simulink model "Simulation_Robotinos"  (R2017b)
settings: Solver=FixedStepAuto  StartTime=0.0  StopTime=100.0  FixedStep=0.005  RelTol=1e-3
InitFcn:
  | dt=0.005;
libraries: simulink x15
(part 1 of 4)
settings Model: Creator=Robin  LastModifiedBy=Robin

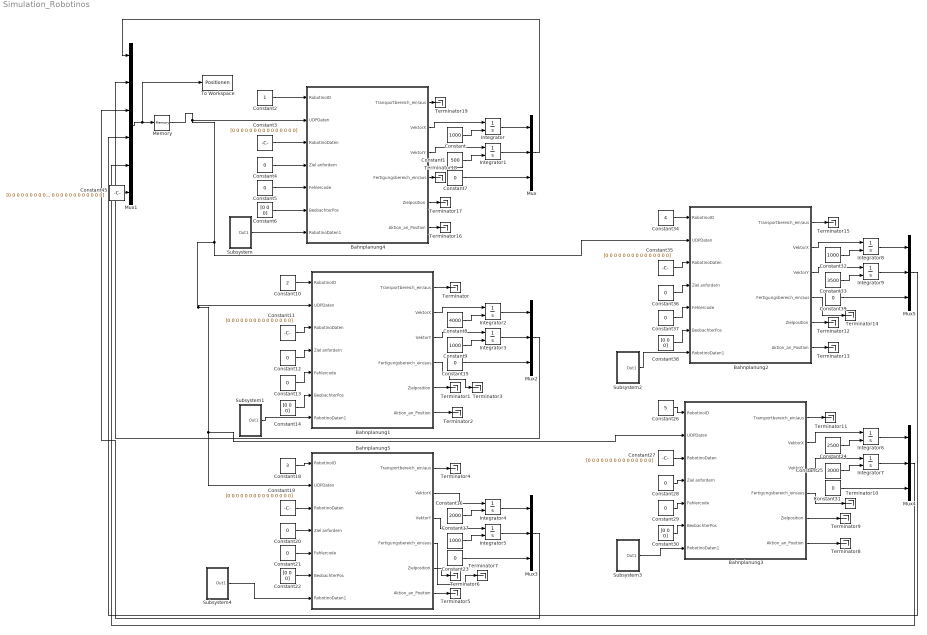
== system Simulation_Robotinos ==
  Bahnplanung1 : Subsystem
  Bahnplanung2 : Subsystem
  Bahnplanung3 : Subsystem
  Bahnplanung4 : Subsystem
  Bahnplanung5 : Subsystem
  Constant{,9,17,32} (4 alike) : Constant  Value=1000
  Constant1 : Constant  Value=500
  Constant10 : Constant  Value=2
  Constant{3,11,19,27,35} (5 alike) : Constant  Value=[0 0 0 0 0 0 0 0 0 0 0 0 0 0 0]
  Constant{4..5,7,12..13,15,20..21,23,28..29,31,36..37,39} (15 alike) : Constant  Value=0
  Constant{6,14,22,30,38} (5 alike) : Constant  Value=[0 0 0]
  Constant16 : Constant  Value=2000
  Constant18 : Constant  Value=3
  Constant2 : Constant
  Constant24 : Constant  Value=2500
  Constant25 : Constant  Value=3000
  Constant26 : Constant  Value=5
  Constant33 : Constant  Value=3500
  Constant34 : Constant  Value=4
  Constant45 : Constant  Value=[0 0 0 0 0 0 0 0 0 0 0 0 0 0 0 0 0 0 0 0 0 0 0 0 0 0 0 0 0 0 0 0 0 0 0 0 0 0 0 0 0]
  Constant8 : Constant  Value=4000
  Integrator{,1..9} (10 alike) : Integrator  InitialConditionSource=external
  Memory : Memory
  Mux{,2..5} (5 alike) : Mux  Inputs=3
  Mux1 : Mux  Inputs=6
  Subsystem : Subsystem
  Subsystem1 : Subsystem
  Subsystem2 : Subsystem
  Subsystem3 : Subsystem
  Subsystem4 : Subsystem
  Terminator{,1..19} (20 alike) : Terminator
  To Workspace : ToWorkspace  VariableName=Positionen  SaveFormat=Timeseries  SampleTime=-1
  wires:
  Bahnplanung4/3("VektorY ") -> Integrator1/1
  Bahnplanung4/2(VektorX) -> Integrator/1
  Constant/1 -> Integrator/2
  Constant1/1 -> Integrator1/2
  Integrator1/1 -> Mux/2
  Constant2/1 -> Bahnplanung4/1(RobotinoID)
  Constant3/1 -> Bahnplanung4/3(RobotinoDaten)
  Constant4/1 -> Bahnplanung4/4(Ziel anfordern)
  Constant5/1 -> Bahnplanung4/5(Fehlercode)
  Constant6/1 -> Bahnplanung4/6(BeobachterPos)
  Constant7/1 -> Mux/3
  Constant15/1 -> Mux2/3
  Constant13/1 -> Bahnplanung1/5(Fehlercode)
  Constant10/1 -> Bahnplanung1/1(RobotinoID)
  Constant8/1 -> Integrator2/2
  Bahnplanung1/3("VektorY ") -> Integrator3/1
  Constant12/1 -> Bahnplanung1/4(Ziel anfordern)
  Bahnplanung1/2(VektorX) -> Integrator2/1
  Constant9/1 -> Integrator3/2
  Integrator3/1 -> Mux2/2
  Integrator2/1 -> Mux2/1
  Constant11/1 -> Bahnplanung1/3(RobotinoDaten)
  Constant14/1 -> Bahnplanung1/6(BeobachterPos)
  Constant23/1 -> Mux3/3
  Constant21/1 -> Bahnplanung5/5(Fehlercode)
  Constant16/1 -> Integrator4/2
  Constant20/1 -> Bahnplanung5/4(Ziel anfordern)
  Constant17/1 -> Integrator5/2
  Integrator5/1 -> Mux3/2
  Integrator4/1 -> Mux3/1
  Constant19/1 -> Bahnplanung5/3(RobotinoDaten)
  Constant22/1 -> Bahnplanung5/6(BeobachterPos)
  Constant31/1 -> Mux4/3
  Constant29/1 -> Bahnplanung3/5(Fehlercode)
  Constant26/1 -> Bahnplanung3/1(RobotinoID)
  Constant24/1 -> Integrator6/2
  Constant28/1 -> Bahnplanung3/4(Ziel anfordern)
  Constant25/1 -> Integrator7/2
  Integrator7/1 -> Mux4/2
  Integrator6/1 -> Mux4/1
  Constant27/1 -> Bahnplanung3/3(RobotinoDaten)
  Constant30/1 -> Bahnplanung3/6(BeobachterPos)
  Constant39/1 -> Mux5/3
  Constant37/1 -> Bahnplanung2/5(Fehlercode)
  Constant34/1 -> Bahnplanung2/1(RobotinoID)
  Constant32/1 -> Integrator8/2
  Constant36/1 -> Bahnplanung2/4(Ziel anfordern)
  Memory/1 -> Bahnplanung2/2(UDPDaten), Bahnplanung1/2(UDPDaten), Bahnplanung5/2(UDPDaten), Bahnplanung3/2(UDPDaten), Bahnplanung4/2(UDPDaten)
  Constant33/1 -> Integrator9/2
  Integrator9/1 -> Mux5/2
  Integrator8/1 -> Mux5/1
  Constant35/1 -> Bahnplanung2/3(RobotinoDaten)
  Constant38/1 -> Bahnplanung2/6(BeobachterPos)
  Mux/1 -> Mux1/1
  Mux2/1 -> Mux1/2
  Mux3/1 -> Mux1/3
  Mux5/1 -> Mux1/4
  Mux4/1 -> Mux1/5
  Constant18/1 -> Bahnplanung5/1(RobotinoID)
  Subsystem4/1(Out1) -> Bahnplanung5/7(RobotinoDaten1)
  Subsystem1/1(Out1) -> Bahnplanung1/7(RobotinoDaten1)
  Subsystem3/1(Out1) -> Bahnplanung3/7(RobotinoDaten1)
  Subsystem2/1(Out1) -> Bahnplanung2/7(RobotinoDaten1)
  Mux1/1 -> To Workspace/1, Memory/1
  Constant45/1 -> Mux1/6
  Bahnplanung1/1(Transportbereich_ein/aus) -> Terminator/1
  Bahnplanung1/5(Zielposition) -> Terminator1/1
  Bahnplanung1/6(Aktion_an_Position) -> Terminator2/1
  Bahnplanung1/4(Fertigungsbereich_ein/aus) -> Terminator3/1
  Bahnplanung5/1(Transportbereich_ein/aus) -> Terminator4/1
  Bahnplanung5/6(Aktion_an_Position) -> Terminator5/1
  Bahnplanung5/5(Zielposition) -> Terminator6/1
  Bahnplanung5/4(Fertigungsbereich_ein/aus) -> Terminator7/1
  Bahnplanung3/5(Zielposition) -> Terminator9/1
  Bahnplanung3/6(Aktion_an_Position) -> Terminator8/1
  Bahnplanung3/4(Fertigungsbereich_ein/aus) -> Terminator10/1
  Bahnplanung3/1(Transportbereich_ein/aus) -> Terminator11/1
  Bahnplanung2/5(Zielposition) -> Terminator12/1
  Bahnplanung2/6(Aktion_an_Position) -> Terminator13/1
  Bahnplanung2/4(Fertigungsbereich_ein/aus) -> Terminator14/1
  Bahnplanung2/1(Transportbereich_ein/aus) -> Terminator15/1
  Bahnplanung4/6(Aktion_an_Position) -> Terminator16/1
  Bahnplanung4/5(Zielposition) -> Terminator17/1
  Bahnplanung4/4(Fertigungsbereich_ein/aus) -> Terminator18/1
  Bahnplanung4/1(Transportbereich_ein/aus) -> Terminator19/1
  Subsystem/1(Out1) -> Bahnplanung4/7(RobotinoDaten1)
  Integrator/1 -> Mux/1
  Bahnplanung5/2(VektorX) -> Integrator4/1
  Bahnplanung5/3("VektorY ") -> Integrator5/1
  Bahnplanung2/2(VektorX) -> Integrator8/1
  Bahnplanung2/3("VektorY ") -> Integrator9/1
  Bahnplanung3/2(VektorX) -> Integrator6/1
  Bahnplanung3/3("VektorY ") -> Integrator7/1

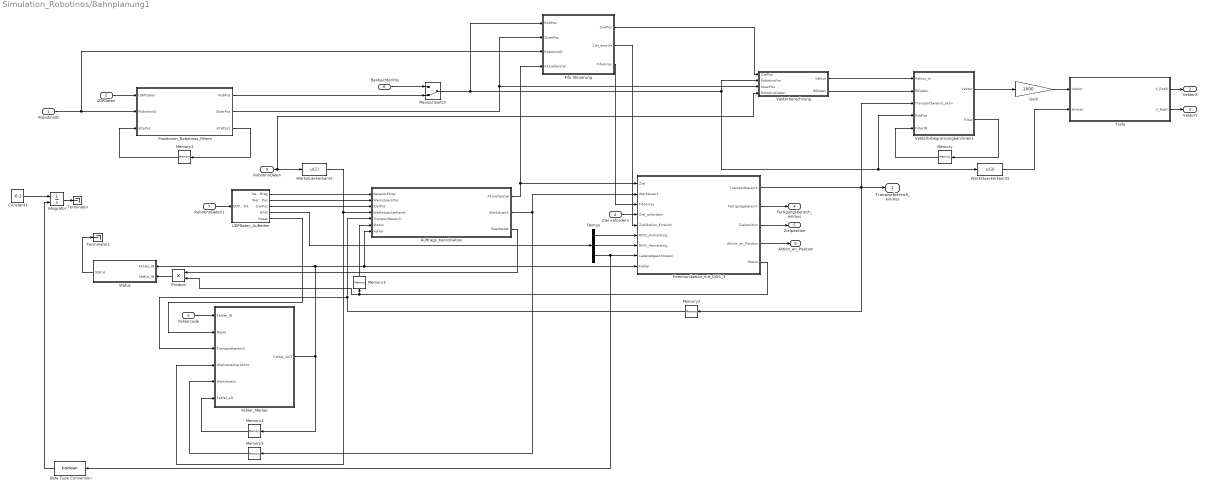
== system Simulation_Robotinos/Bahnplanung1 ==
  RobotinoID : Inport
  UDPDaten : Inport  Port=2  PortDimensions=56
  RobotinoDaten : Inport  Port=3
  Ziel anfordern : Inport  Port=4
  Fehlercode : Inport  Port=5
  BeobachterPos : Inport  Port=6
  RobotinoDaten1 : Inport  Port=7
  Auftrags_Koordination : Stateflow chart  TreatAsAtomicUnit=on
  Constant1 : Constant  Value=-0.2
  Data Type Conversion : DataTypeConversion  OutDataTypeStr=boolean
  Demux : Demux  Outputs=3
  Fehler_Merker : MATLAB Function  TreatAsAtomicUnit=on
  Fifo Steuerung : Subsystem
  Gain : Gain  Gain=-1000
  Integrator : Integrator  ExternalReset=rising  InitialCondition=100  LimitOutput=on  UpperSaturationLimit=100  LowerSaturationLimit=0
  Kommunikation_mit_GW1_3 : Stateflow chart  TreatAsAtomicUnit=on
  Manual Switch : ManualSwitch  CurrentSetting=0
  Memory{,1..5} (6 alike) : Memory
  Positionen_Robotinos_Filtern : MATLAB Function  TreatAsAtomicUnit=on
  Product : Product
  Status : MATLAB Function  TreatAsAtomicUnit=on
  Terminator : Terminator
  Terminator1 : Terminator
  Trafo : MATLAB Function  Tag=Transformation_Global_auf_lokal  TreatAsAtomicUnit=on
  UDPDaten_Aufteilen : Subsystem
  Vektorberechnung : Subsystem
  Vektorbrbegrenzungberchnen1 : MATLAB Function  TreatAsAtomicUnit=on
  Werkstueckerkannt : Fcn  Expr=u(1)
  Werkstueckerkannt1 : Fcn  Expr=u(3)
  Transportbereich_ein/aus : Outport
  VektorX : Outport  Port=2  OutDataTypeStr=double  PortDimensions=1
  "VektorY " : Outport  Port=3  OutDataTypeStr=double  PortDimensions=1
  Fertigungsbereich_ein/aus : Outport  Port=4
  Zielposition : Outport  Port=5
  Aktion_an_Position : Outport  Port=6
  wires:
  Vektorberechnung/2(IRDaten) -> Vektorbrbegrenzungberchnen1/2(IRDaten)
  Auftrags_Koordination/2(Werkstueck) -> Memory5/1, Kommunikation_mit_GW1_3/2(Werkstueck)
  Memory3/1 -> Auftrags_Koordination/6(Status)
  Kommunikation_mit_GW1_3/5(Status) -> Product/2, Memory3/1
  RobotinoID/1 -> Positionen_Robotinos_Filtern/2(RobotinoID), Fifo Steuerung/3(RobotinoID)
  UDPDaten/1 -> Positionen_Robotinos_Filtern/1(UDPDaten)
  Positionen_Robotinos_Filtern/2(StoerPos) -> Vektorberechnung/3(StoerPos), Fifo Steuerung/2(StoerPos)
  RobotinoDaten/1 -> Werkstueckerkannt/1, Vektorberechnung/4(RobotinoDaten)
  Kommunikation_mit_GW1_3/3(Zielposition) -> Zielposition/1
  Kommunikation_mit_GW1_3/4(Aktion_an_Position) -> Aktion_an_Position/1
  Kommunikation_mit_GW1_3/2(Fertigungsbereich) -> Fertigungsbereich_ein/aus/1
  Kommunikation_mit_GW1_3/1(Transportbereich) -> Transportbereich_ein/aus/1, Vektorbrbegrenzungberchnen1/3(Transportbereich_aktiv), Memory2/1
  RobotinoDaten1/1 -> UDPDaten_Aufteilen/1(UDP_GW1)
  UDPDaten_Aufteilen/2(WerkstueckPos) -> Auftrags_Koordination/2(WerkstueckPos)
  UDPDaten_Aufteilen/3(ZielPos) -> Auftrags_Koordination/3(ZielPos)
  Auftrags_Koordination/1(AktuellesZiel) -> Fifo Steuerung/4(AktuellesZiel), Kommunikation_mit_GW1_3/1(Ziel)
  UDPDaten_Aufteilen/1(NeuerAuftrag) -> Auftrags_Koordination/1(NeuerAuftrag)
  Werkstueckerkannt/1 -> Auftrags_Koordination/4(Werkstueckerkannt), Fehler_Merker/4(Werkstueckerkannt)
  Vektorbrbegrenzungberchnen1/1(Vektor) -> Gain/1
  Gain/1 -> Trafo/1(Vektor)
  Manual Switch/1 -> Vektorberechnung/2(RobotinoPos), Vektorbrbegrenzungberchnen1/4(RobPos), Werkstueckerkannt1/1, Fifo Steuerung/1(RobPos)
  Vektorberechnung/1(Vektor) -> Vektorbrbegrenzungberchnen1/1(Vektor_In)
  Fifo Steuerung/1(ZielPos) -> Vektorberechnung/1(ZielPos)
  Memory2/1 -> Auftrags_Koordination/5(Transportbereich), Fehler_Merker/3(Transportbereich)
  Positionen_Robotinos_Filtern/1(RobPos) -> Manual Switch/2
  Trafo/1(V_RobX) -> VektorX/1
  Trafo/2(V_RobY) -> "VektorY "/1
  BeobachterPos/1 -> Manual Switch/1
  Werkstueckerkannt1/1 -> Trafo/2(Winkel)
  Auftrags_Koordination/3(Bearbeitet) -> Product/1
  UDPDaten_Aufteilen/4(RFID) -> Demux/1
  Fifo Steuerung/3("FifoArray ") -> Kommunikation_mit_GW1_3/3(FifoArray)
  Ziel anfordern/1 -> Kommunikation_mit_GW1_3/4(Ziel_anfordern)
  Fifo Steuerung/2(Ziel_ereciht) -> Kommunikation_mit_GW1_3/5(ZielStation_Erreicht)
  Demux/1 -> Kommunikation_mit_GW1_3/6(RFID_Anmeldung)
  Demux/2 -> Kommunikation_mit_GW1_3/7(RFID_Abmeldung)
  Vektorbrbegrenzungberchnen1/2(Filter) -> Memory/1
  Memory/1 -> Vektorbrbegrenzungberchnen1/5(FilterIN)
  Positionen_Robotinos_Filtern/3(altePos1) -> Memory1/1
  Memory1/1 -> Positionen_Robotinos_Filtern/3(altePos)
  Demux/3 -> Kommunikation_mit_GW1_3/8(Ladenabgeschlossen), Data Type Conversion/1
  Fehlercode/1 -> Fehler_Merker/1(Fehler_IN)
  Constant1/1 -> Integrator/1
  Data Type Conversion/1 -> Integrator/2
  Product/1 -> Status/2(Status_IN)
  UDPDaten_Aufteilen/5(Reset) -> Fehler_Merker/2(Reset)
  Memory4/1 -> Fehler_Merker/6(Fehler_alt)
  Fehler_Merker/1(Fehler_OUT) -> Status/1(Fehler_IN), Kommunikation_mit_GW1_3/9(Fehler), Auftrags_Koordination/7(Fehler), Memory4/1
  Memory5/1 -> Fehler_Merker/5(Werkstueck)
  Integrator/1 -> Terminator/1
  Status/1(Status) -> Terminator1/1

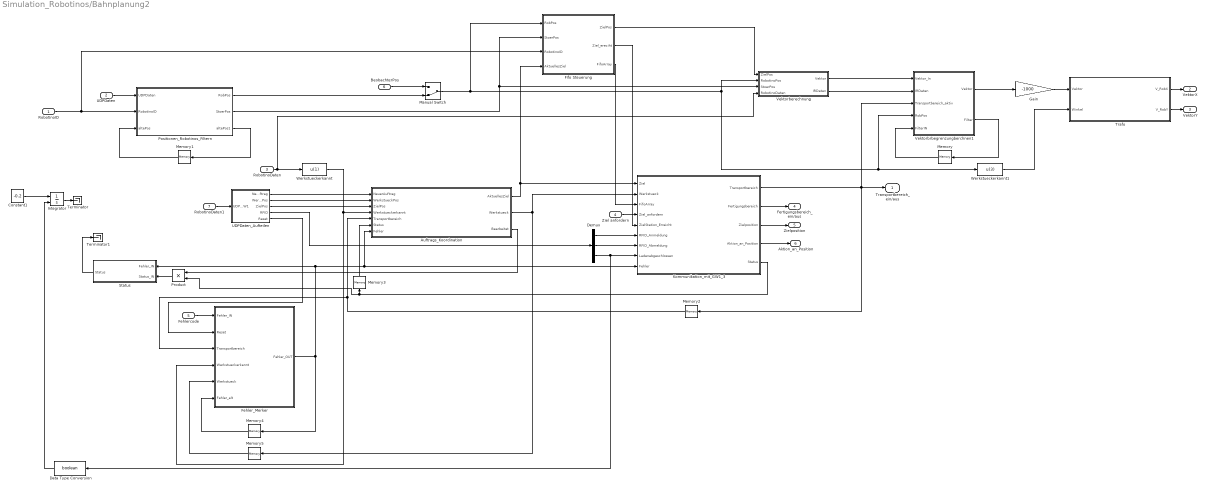
== system Simulation_Robotinos/Bahnplanung2 ==
  RobotinoID : Inport
  UDPDaten : Inport  Port=2  PortDimensions=56
  RobotinoDaten : Inport  Port=3
  Ziel anfordern : Inport  Port=4
  Fehlercode : Inport  Port=5
  BeobachterPos : Inport  Port=6
  RobotinoDaten1 : Inport  Port=7
  Auftrags_Koordination : Stateflow chart  TreatAsAtomicUnit=on
  Constant1 : Constant  Value=-0.2
  Data Type Conversion : DataTypeConversion  OutDataTypeStr=boolean
  Demux : Demux  Outputs=3
  Fehler_Merker : MATLAB Function  TreatAsAtomicUnit=on
  Fifo Steuerung : Subsystem
  Gain : Gain  Gain=-1000
  Integrator : Integrator  ExternalReset=rising  InitialCondition=100  LimitOutput=on  UpperSaturationLimit=100  LowerSaturationLimit=0
  Kommunikation_mit_GW1_3 : Stateflow chart  TreatAsAtomicUnit=on
  Manual Switch : ManualSwitch  CurrentSetting=0
  Memory{,1..5} (6 alike) : Memory
  Positionen_Robotinos_Filtern : MATLAB Function  TreatAsAtomicUnit=on
  Product : Product
  Status : MATLAB Function  TreatAsAtomicUnit=on
  Terminator : Terminator
  Terminator1 : Terminator
  Trafo : MATLAB Function  Tag=Transformation_Global_auf_lokal  TreatAsAtomicUnit=on
  UDPDaten_Aufteilen : Subsystem
  Vektorberechnung : Subsystem
  Vektorbrbegrenzungberchnen1 : MATLAB Function  TreatAsAtomicUnit=on
  Werkstueckerkannt : Fcn  Expr=u(1)
  Werkstueckerkannt1 : Fcn  Expr=u(3)
  Transportbereich_ein/aus : Outport
  VektorX : Outport  Port=2  OutDataTypeStr=double  PortDimensions=1
  "VektorY " : Outport  Port=3  OutDataTypeStr=double  PortDimensions=1
  Fertigungsbereich_ein/aus : Outport  Port=4
  Zielposition : Outport  Port=5
  Aktion_an_Position : Outport  Port=6
  wires:
  Status/1(Status) -> Terminator1/1
  Integrator/1 -> Terminator/1
  Memory5/1 -> Fehler_Merker/5(Werkstueck)
  Fehler_Merker/1(Fehler_OUT) -> Memory4/1, Auftrags_Koordination/7(Fehler), Kommunikation_mit_GW1_3/9(Fehler), Status/1(Fehler_IN)
  Memory4/1 -> Fehler_Merker/6(Fehler_alt)
  UDPDaten_Aufteilen/5(Reset) -> Fehler_Merker/2(Reset)
  Product/1 -> Status/2(Status_IN)
  Data Type Conversion/1 -> Integrator/2
  Constant1/1 -> Integrator/1
  Fehlercode/1 -> Fehler_Merker/1(Fehler_IN)
  Demux/3 -> Data Type Conversion/1, Kommunikation_mit_GW1_3/8(Ladenabgeschlossen)
  Memory1/1 -> Positionen_Robotinos_Filtern/3(altePos)
  Positionen_Robotinos_Filtern/3(altePos1) -> Memory1/1
  Memory/1 -> Vektorbrbegrenzungberchnen1/5(FilterIN)
  Vektorbrbegrenzungberchnen1/2(Filter) -> Memory/1
  Demux/2 -> Kommunikation_mit_GW1_3/7(RFID_Abmeldung)
  Demux/1 -> Kommunikation_mit_GW1_3/6(RFID_Anmeldung)
  Fifo Steuerung/2(Ziel_ereciht) -> Kommunikation_mit_GW1_3/5(ZielStation_Erreicht)
  Ziel anfordern/1 -> Kommunikation_mit_GW1_3/4(Ziel_anfordern)
  Fifo Steuerung/3("FifoArray ") -> Kommunikation_mit_GW1_3/3(FifoArray)
  UDPDaten_Aufteilen/4(RFID) -> Demux/1
  Auftrags_Koordination/3(Bearbeitet) -> Product/1
  Werkstueckerkannt1/1 -> Trafo/2(Winkel)
  BeobachterPos/1 -> Manual Switch/1
  Trafo/2(V_RobY) -> "VektorY "/1
  Trafo/1(V_RobX) -> VektorX/1
  Positionen_Robotinos_Filtern/1(RobPos) -> Manual Switch/2
  Memory2/1 -> Fehler_Merker/3(Transportbereich), Auftrags_Koordination/5(Transportbereich)
  Fifo Steuerung/1(ZielPos) -> Vektorberechnung/1(ZielPos)
  Vektorberechnung/1(Vektor) -> Vektorbrbegrenzungberchnen1/1(Vektor_In)
  Manual Switch/1 -> Fifo Steuerung/1(RobPos), Werkstueckerkannt1/1, Vektorbrbegrenzungberchnen1/4(RobPos), Vektorberechnung/2(RobotinoPos)
  Gain/1 -> Trafo/1(Vektor)
  Vektorbrbegrenzungberchnen1/1(Vektor) -> Gain/1
  Werkstueckerkannt/1 -> Fehler_Merker/4(Werkstueckerkannt), Auftrags_Koordination/4(Werkstueckerkannt)
  UDPDaten_Aufteilen/1(NeuerAuftrag) -> Auftrags_Koordination/1(NeuerAuftrag)
  Auftrags_Koordination/1(AktuellesZiel) -> Kommunikation_mit_GW1_3/1(Ziel), Fifo Steuerung/4(AktuellesZiel)
  UDPDaten_Aufteilen/3(ZielPos) -> Auftrags_Koordination/3(ZielPos)
  UDPDaten_Aufteilen/2(WerkstueckPos) -> Auftrags_Koordination/2(WerkstueckPos)
  RobotinoDaten1/1 -> UDPDaten_Aufteilen/1(UDP_GW1)
  Kommunikation_mit_GW1_3/1(Transportbereich) -> Memory2/1, Vektorbrbegrenzungberchnen1/3(Transportbereich_aktiv), Transportbereich_ein/aus/1
  Kommunikation_mit_GW1_3/2(Fertigungsbereich) -> Fertigungsbereich_ein/aus/1
  Kommunikation_mit_GW1_3/4(Aktion_an_Position) -> Aktion_an_Position/1
  Kommunikation_mit_GW1_3/3(Zielposition) -> Zielposition/1
  RobotinoDaten/1 -> Vektorberechnung/4(RobotinoDaten), Werkstueckerkannt/1
  Positionen_Robotinos_Filtern/2(StoerPos) -> Fifo Steuerung/2(StoerPos), Vektorberechnung/3(StoerPos)
  UDPDaten/1 -> Positionen_Robotinos_Filtern/1(UDPDaten)
  RobotinoID/1 -> Fifo Steuerung/3(RobotinoID), Positionen_Robotinos_Filtern/2(RobotinoID)
  Kommunikation_mit_GW1_3/5(Status) -> Memory3/1, Product/2
  Memory3/1 -> Auftrags_Koordination/6(Status)
  Auftrags_Koordination/2(Werkstueck) -> Kommunikation_mit_GW1_3/2(Werkstueck), Memory5/1
  Vektorberechnung/2(IRDaten) -> Vektorbrbegrenzungberchnen1/2(IRDaten)

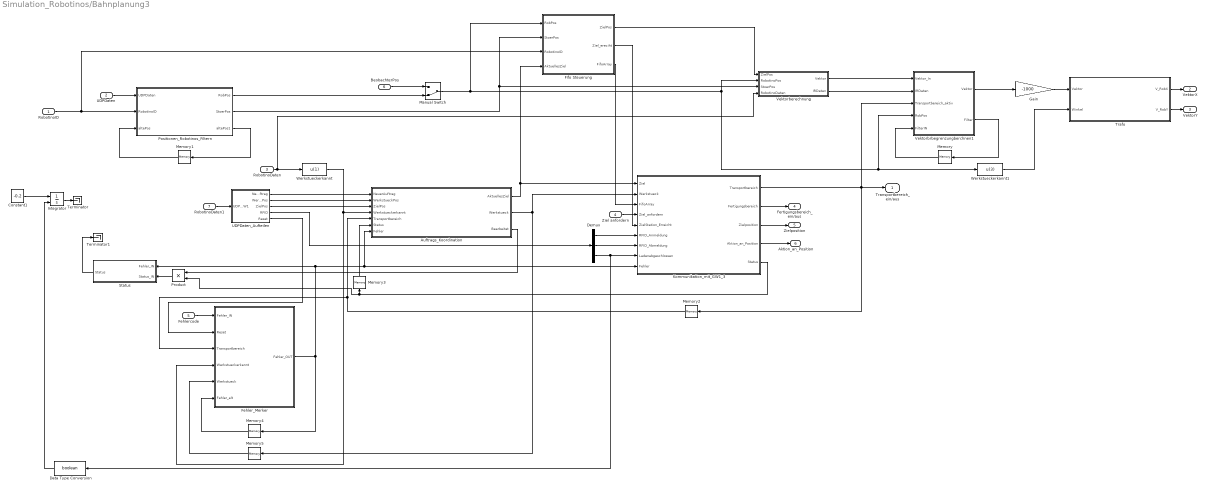
== system Simulation_Robotinos/Bahnplanung3 ==
  RobotinoID : Inport
  UDPDaten : Inport  Port=2  PortDimensions=56
  RobotinoDaten : Inport  Port=3
  Ziel anfordern : Inport  Port=4
  Fehlercode : Inport  Port=5
  BeobachterPos : Inport  Port=6
  RobotinoDaten1 : Inport  Port=7
  Auftrags_Koordination : Stateflow chart  TreatAsAtomicUnit=on
  Constant1 : Constant  Value=-0.2
  Data Type Conversion : DataTypeConversion  OutDataTypeStr=boolean
  Demux : Demux  Outputs=3
  Fehler_Merker : MATLAB Function  TreatAsAtomicUnit=on
  Fifo Steuerung : Subsystem
  Gain : Gain  Gain=-1000
  Integrator : Integrator  ExternalReset=rising  InitialCondition=100  LimitOutput=on  UpperSaturationLimit=100  LowerSaturationLimit=0
  Kommunikation_mit_GW1_3 : Stateflow chart  TreatAsAtomicUnit=on
  Manual Switch : ManualSwitch  CurrentSetting=0
  Memory{,1..5} (6 alike) : Memory
  Positionen_Robotinos_Filtern : MATLAB Function  TreatAsAtomicUnit=on
  Product : Product
  Status : MATLAB Function  TreatAsAtomicUnit=on
  Terminator : Terminator
  Terminator1 : Terminator
  Trafo : MATLAB Function  Tag=Transformation_Global_auf_lokal  TreatAsAtomicUnit=on
  UDPDaten_Aufteilen : Subsystem
  Vektorberechnung : Subsystem
  Vektorbrbegrenzungberchnen1 : MATLAB Function  TreatAsAtomicUnit=on
  Werkstueckerkannt : Fcn  Expr=u(1)
  Werkstueckerkannt1 : Fcn  Expr=u(3)
  Transportbereich_ein/aus : Outport
  VektorX : Outport  Port=2  OutDataTypeStr=double  PortDimensions=1
  "VektorY " : Outport  Port=3  OutDataTypeStr=double  PortDimensions=1
  Fertigungsbereich_ein/aus : Outport  Port=4
  Zielposition : Outport  Port=5
  Aktion_an_Position : Outport  Port=6
  wires:
  Vektorberechnung/2(IRDaten) -> Vektorbrbegrenzungberchnen1/2(IRDaten)
  Auftrags_Koordination/2(Werkstueck) -> Memory5/1, Kommunikation_mit_GW1_3/2(Werkstueck)
  Memory3/1 -> Auftrags_Koordination/6(Status)
  Kommunikation_mit_GW1_3/5(Status) -> Product/2, Memory3/1
  RobotinoID/1 -> Positionen_Robotinos_Filtern/2(RobotinoID), Fifo Steuerung/3(RobotinoID)
  UDPDaten/1 -> Positionen_Robotinos_Filtern/1(UDPDaten)
  Positionen_Robotinos_Filtern/2(StoerPos) -> Vektorberechnung/3(StoerPos), Fifo Steuerung/2(StoerPos)
  RobotinoDaten/1 -> Werkstueckerkannt/1, Vektorberechnung/4(RobotinoDaten)
  Kommunikation_mit_GW1_3/3(Zielposition) -> Zielposition/1
  Kommunikation_mit_GW1_3/4(Aktion_an_Position) -> Aktion_an_Position/1
  Kommunikation_mit_GW1_3/2(Fertigungsbereich) -> Fertigungsbereich_ein/aus/1
  Kommunikation_mit_GW1_3/1(Transportbereich) -> Transportbereich_ein/aus/1, Vektorbrbegrenzungberchnen1/3(Transportbereich_aktiv), Memory2/1
  RobotinoDaten1/1 -> UDPDaten_Aufteilen/1(UDP_GW1)
  UDPDaten_Aufteilen/2(WerkstueckPos) -> Auftrags_Koordination/2(WerkstueckPos)
  UDPDaten_Aufteilen/3(ZielPos) -> Auftrags_Koordination/3(ZielPos)
  Auftrags_Koordination/1(AktuellesZiel) -> Fifo Steuerung/4(AktuellesZiel), Kommunikation_mit_GW1_3/1(Ziel)
  UDPDaten_Aufteilen/1(NeuerAuftrag) -> Auftrags_Koordination/1(NeuerAuftrag)
  Werkstueckerkannt/1 -> Auftrags_Koordination/4(Werkstueckerkannt), Fehler_Merker/4(Werkstueckerkannt)
  Vektorbrbegrenzungberchnen1/1(Vektor) -> Gain/1
  Gain/1 -> Trafo/1(Vektor)
  Manual Switch/1 -> Vektorberechnung/2(RobotinoPos), Vektorbrbegrenzungberchnen1/4(RobPos), Werkstueckerkannt1/1, Fifo Steuerung/1(RobPos)
  Vektorberechnung/1(Vektor) -> Vektorbrbegrenzungberchnen1/1(Vektor_In)
  Fifo Steuerung/1(ZielPos) -> Vektorberechnung/1(ZielPos)
  Memory2/1 -> Auftrags_Koordination/5(Transportbereich), Fehler_Merker/3(Transportbereich)
  Positionen_Robotinos_Filtern/1(RobPos) -> Manual Switch/2
  Trafo/1(V_RobX) -> VektorX/1
  Trafo/2(V_RobY) -> "VektorY "/1
  BeobachterPos/1 -> Manual Switch/1
  Werkstueckerkannt1/1 -> Trafo/2(Winkel)
  Auftrags_Koordination/3(Bearbeitet) -> Product/1
  UDPDaten_Aufteilen/4(RFID) -> Demux/1
  Fifo Steuerung/3("FifoArray ") -> Kommunikation_mit_GW1_3/3(FifoArray)
  Ziel anfordern/1 -> Kommunikation_mit_GW1_3/4(Ziel_anfordern)
  Fifo Steuerung/2(Ziel_ereciht) -> Kommunikation_mit_GW1_3/5(ZielStation_Erreicht)
  Demux/1 -> Kommunikation_mit_GW1_3/6(RFID_Anmeldung)
  Demux/2 -> Kommunikation_mit_GW1_3/7(RFID_Abmeldung)
  Vektorbrbegrenzungberchnen1/2(Filter) -> Memory/1
  Memory/1 -> Vektorbrbegrenzungberchnen1/5(FilterIN)
  Positionen_Robotinos_Filtern/3(altePos1) -> Memory1/1
  Memory1/1 -> Positionen_Robotinos_Filtern/3(altePos)
  Demux/3 -> Kommunikation_mit_GW1_3/8(Ladenabgeschlossen), Data Type Conversion/1
  Fehlercode/1 -> Fehler_Merker/1(Fehler_IN)
  Constant1/1 -> Integrator/1
  Data Type Conversion/1 -> Integrator/2
  Product/1 -> Status/2(Status_IN)
  UDPDaten_Aufteilen/5(Reset) -> Fehler_Merker/2(Reset)
  Memory4/1 -> Fehler_Merker/6(Fehler_alt)
  Fehler_Merker/1(Fehler_OUT) -> Status/1(Fehler_IN), Kommunikation_mit_GW1_3/9(Fehler), Auftrags_Koordination/7(Fehler), Memory4/1
  Memory5/1 -> Fehler_Merker/5(Werkstueck)
  Integrator/1 -> Terminator/1
  Status/1(Status) -> Terminator1/1

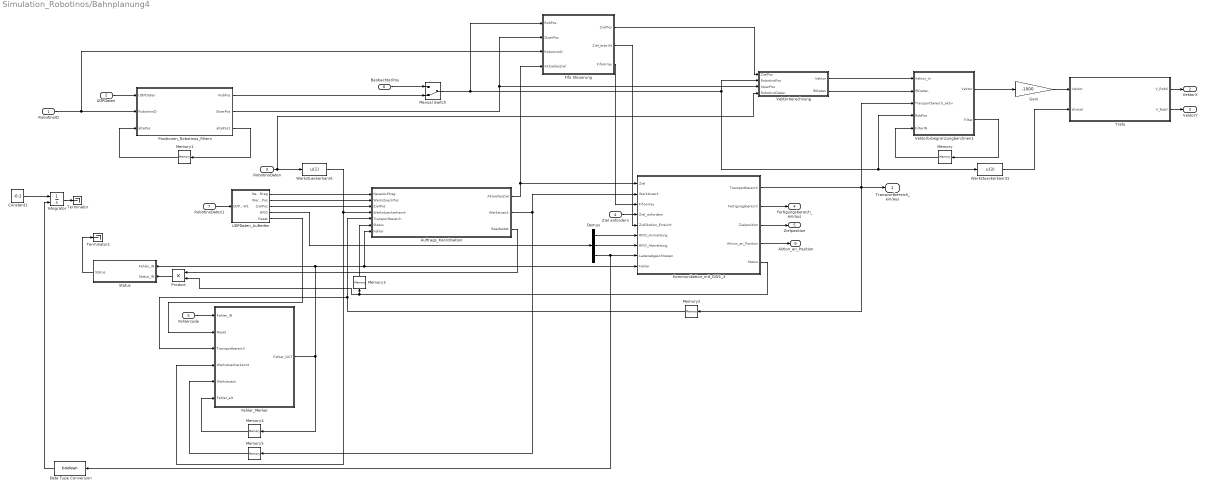
== system Simulation_Robotinos/Bahnplanung4 ==
  RobotinoID : Inport
  UDPDaten : Inport  Port=2  PortDimensions=56
  RobotinoDaten : Inport  Port=3
  Ziel anfordern : Inport  Port=4
  Fehlercode : Inport  Port=5
  BeobachterPos : Inport  Port=6
  RobotinoDaten1 : Inport  Port=7
  Auftrags_Koordination : Stateflow chart  TreatAsAtomicUnit=on
  Constant1 : Constant  Value=-0.2
  Data Type Conversion : DataTypeConversion  OutDataTypeStr=boolean
  Demux : Demux  Outputs=3
  Fehler_Merker : MATLAB Function  TreatAsAtomicUnit=on
  Fifo Steuerung : Subsystem
  Gain : Gain  Gain=-1000
  Integrator : Integrator  ExternalReset=rising  InitialCondition=100  LimitOutput=on  UpperSaturationLimit=100  LowerSaturationLimit=0
  Kommunikation_mit_GW1_3 : Stateflow chart  TreatAsAtomicUnit=on
  Manual Switch : ManualSwitch  CurrentSetting=0
  Memory{,1..5} (6 alike) : Memory
  Positionen_Robotinos_Filtern : MATLAB Function  TreatAsAtomicUnit=on
  Product : Product
  Status : MATLAB Function  TreatAsAtomicUnit=on
  Terminator : Terminator
  Terminator1 : Terminator
  Trafo : MATLAB Function  Tag=Transformation_Global_auf_lokal  TreatAsAtomicUnit=on
  UDPDaten_Aufteilen : Subsystem
  Vektorberechnung : Subsystem
  Vektorbrbegrenzungberchnen1 : MATLAB Function  TreatAsAtomicUnit=on
  Werkstueckerkannt : Fcn  Expr=u(1)
  Werkstueckerkannt1 : Fcn  Expr=u(3)
  Transportbereich_ein/aus : Outport
  VektorX : Outport  Port=2  OutDataTypeStr=double  PortDimensions=1
  "VektorY " : Outport  Port=3  OutDataTypeStr=double  PortDimensions=1
  Fertigungsbereich_ein/aus : Outport  Port=4
  Zielposition : Outport  Port=5
  Aktion_an_Position : Outport  Port=6
  wires:
  Status/1(Status) -> Terminator1/1
  Integrator/1 -> Terminator/1
  Memory5/1 -> Fehler_Merker/5(Werkstueck)
  Fehler_Merker/1(Fehler_OUT) -> Memory4/1, Auftrags_Koordination/7(Fehler), Kommunikation_mit_GW1_3/9(Fehler), Status/1(Fehler_IN)
  Memory4/1 -> Fehler_Merker/6(Fehler_alt)
  UDPDaten_Aufteilen/5(Reset) -> Fehler_Merker/2(Reset)
  Product/1 -> Status/2(Status_IN)
  Data Type Conversion/1 -> Integrator/2
  Constant1/1 -> Integrator/1
  Fehlercode/1 -> Fehler_Merker/1(Fehler_IN)
  Demux/3 -> Data Type Conversion/1, Kommunikation_mit_GW1_3/8(Ladenabgeschlossen)
  Memory1/1 -> Positionen_Robotinos_Filtern/3(altePos)
  Positionen_Robotinos_Filtern/3(altePos1) -> Memory1/1
  Memory/1 -> Vektorbrbegrenzungberchnen1/5(FilterIN)
  Vektorbrbegrenzungberchnen1/2(Filter) -> Memory/1
  Demux/2 -> Kommunikation_mit_GW1_3/7(RFID_Abmeldung)
  Demux/1 -> Kommunikation_mit_GW1_3/6(RFID_Anmeldung)
  Fifo Steuerung/2(Ziel_ereciht) -> Kommunikation_mit_GW1_3/5(ZielStation_Erreicht)
  Ziel anfordern/1 -> Kommunikation_mit_GW1_3/4(Ziel_anfordern)
  Fifo Steuerung/3("FifoArray ") -> Kommunikation_mit_GW1_3/3(FifoArray)
  UDPDaten_Aufteilen/4(RFID) -> Demux/1
  Auftrags_Koordination/3(Bearbeitet) -> Product/1
  Werkstueckerkannt1/1 -> Trafo/2(Winkel)
  BeobachterPos/1 -> Manual Switch/1
  Trafo/2(V_RobY) -> "VektorY "/1
  Trafo/1(V_RobX) -> VektorX/1
  Positionen_Robotinos_Filtern/1(RobPos) -> Manual Switch/2
  Memory2/1 -> Fehler_Merker/3(Transportbereich), Auftrags_Koordination/5(Transportbereich)
  Fifo Steuerung/1(ZielPos) -> Vektorberechnung/1(ZielPos)
  Vektorberechnung/1(Vektor) -> Vektorbrbegrenzungberchnen1/1(Vektor_In)
  Manual Switch/1 -> Fifo Steuerung/1(RobPos), Werkstueckerkannt1/1, Vektorbrbegrenzungberchnen1/4(RobPos), Vektorberechnung/2(RobotinoPos)
  Gain/1 -> Trafo/1(Vektor)
  Vektorbrbegrenzungberchnen1/1(Vektor) -> Gain/1
  Werkstueckerkannt/1 -> Fehler_Merker/4(Werkstueckerkannt), Auftrags_Koordination/4(Werkstueckerkannt)
  UDPDaten_Aufteilen/1(NeuerAuftrag) -> Auftrags_Koordination/1(NeuerAuftrag)
  Auftrags_Koordination/1(AktuellesZiel) -> Kommunikation_mit_GW1_3/1(Ziel), Fifo Steuerung/4(AktuellesZiel)
  UDPDaten_Aufteilen/3(ZielPos) -> Auftrags_Koordination/3(ZielPos)
  UDPDaten_Aufteilen/2(WerkstueckPos) -> Auftrags_Koordination/2(WerkstueckPos)
  RobotinoDaten1/1 -> UDPDaten_Aufteilen/1(UDP_GW1)
  Kommunikation_mit_GW1_3/1(Transportbereich) -> Memory2/1, Vektorbrbegrenzungberchnen1/3(Transportbereich_aktiv), Transportbereich_ein/aus/1
  Kommunikation_mit_GW1_3/2(Fertigungsbereich) -> Fertigungsbereich_ein/aus/1
  Kommunikation_mit_GW1_3/4(Aktion_an_Position) -> Aktion_an_Position/1
  Kommunikation_mit_GW1_3/3(Zielposition) -> Zielposition/1
  RobotinoDaten/1 -> Vektorberechnung/4(RobotinoDaten), Werkstueckerkannt/1
  Positionen_Robotinos_Filtern/2(StoerPos) -> Fifo Steuerung/2(StoerPos), Vektorberechnung/3(StoerPos)
  UDPDaten/1 -> Positionen_Robotinos_Filtern/1(UDPDaten)
  RobotinoID/1 -> Fifo Steuerung/3(RobotinoID), Positionen_Robotinos_Filtern/2(RobotinoID)
  Kommunikation_mit_GW1_3/5(Status) -> Memory3/1, Product/2
  Memory3/1 -> Auftrags_Koordination/6(Status)
  Auftrags_Koordination/2(Werkstueck) -> Kommunikation_mit_GW1_3/2(Werkstueck), Memory5/1
  Vektorberechnung/2(IRDaten) -> Vektorbrbegrenzungberchnen1/2(IRDaten)

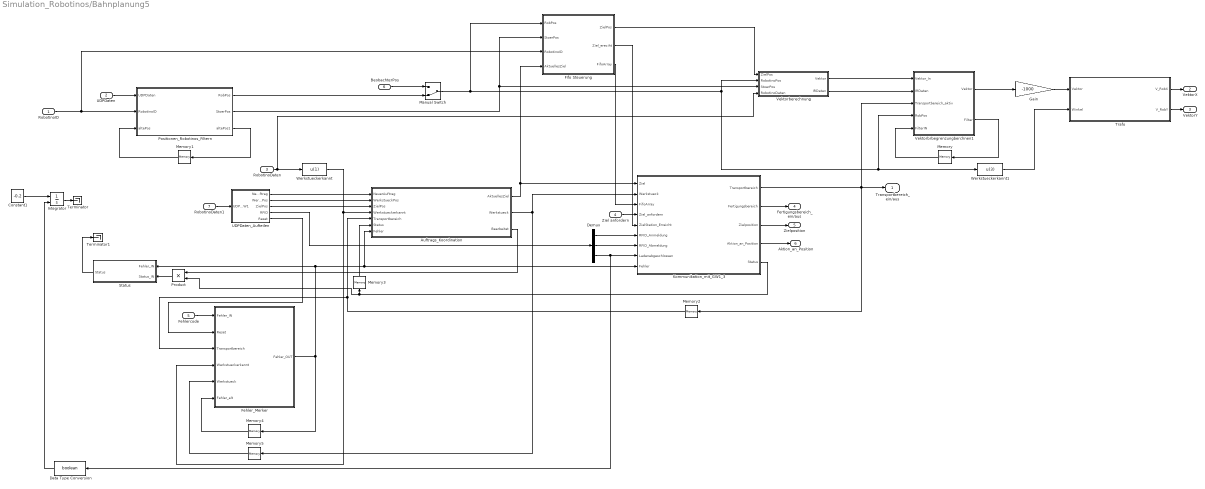
== system Simulation_Robotinos/Bahnplanung5 ==
  RobotinoID : Inport
  UDPDaten : Inport  Port=2  PortDimensions=56
  RobotinoDaten : Inport  Port=3
  Ziel anfordern : Inport  Port=4
  Fehlercode : Inport  Port=5
  BeobachterPos : Inport  Port=6
  RobotinoDaten1 : Inport  Port=7
  Auftrags_Koordination : Stateflow chart  TreatAsAtomicUnit=on
  Constant1 : Constant  Value=-0.2
  Data Type Conversion : DataTypeConversion  OutDataTypeStr=boolean
  Demux : Demux  Outputs=3
  Fehler_Merker : MATLAB Function  TreatAsAtomicUnit=on
  Fifo Steuerung : Subsystem
  Gain : Gain  Gain=-1000
  Integrator : Integrator  ExternalReset=rising  InitialCondition=100  LimitOutput=on  UpperSaturationLimit=100  LowerSaturationLimit=0
  Kommunikation_mit_GW1_3 : Stateflow chart  TreatAsAtomicUnit=on
  Manual Switch : ManualSwitch  CurrentSetting=0
  Memory{,1..5} (6 alike) : Memory
  Positionen_Robotinos_Filtern : MATLAB Function  TreatAsAtomicUnit=on
  Product : Product
  Status : MATLAB Function  TreatAsAtomicUnit=on
  Terminator : Terminator
  Terminator1 : Terminator
  Trafo : MATLAB Function  Tag=Transformation_Global_auf_lokal  TreatAsAtomicUnit=on
  UDPDaten_Aufteilen : Subsystem
  Vektorberechnung : Subsystem
  Vektorbrbegrenzungberchnen1 : MATLAB Function  TreatAsAtomicUnit=on
  Werkstueckerkannt : Fcn  Expr=u(1)
  Werkstueckerkannt1 : Fcn  Expr=u(3)
  Transportbereich_ein/aus : Outport
  VektorX : Outport  Port=2  OutDataTypeStr=double  PortDimensions=1
  "VektorY " : Outport  Port=3  OutDataTypeStr=double  PortDimensions=1
  Fertigungsbereich_ein/aus : Outport  Port=4
  Zielposition : Outport  Port=5
  Aktion_an_Position : Outport  Port=6
  wires:
  Status/1(Status) -> Terminator1/1
  Integrator/1 -> Terminator/1
  Memory5/1 -> Fehler_Merker/5(Werkstueck)
  Fehler_Merker/1(Fehler_OUT) -> Memory4/1, Auftrags_Koordination/7(Fehler), Kommunikation_mit_GW1_3/9(Fehler), Status/1(Fehler_IN)
  Memory4/1 -> Fehler_Merker/6(Fehler_alt)
  UDPDaten_Aufteilen/5(Reset) -> Fehler_Merker/2(Reset)
  Product/1 -> Status/2(Status_IN)
  Data Type Conversion/1 -> Integrator/2
  Constant1/1 -> Integrator/1
  Fehlercode/1 -> Fehler_Merker/1(Fehler_IN)
  Demux/3 -> Data Type Conversion/1, Kommunikation_mit_GW1_3/8(Ladenabgeschlossen)
  Memory1/1 -> Positionen_Robotinos_Filtern/3(altePos)
  Positionen_Robotinos_Filtern/3(altePos1) -> Memory1/1
  Memory/1 -> Vektorbrbegrenzungberchnen1/5(FilterIN)
  Vektorbrbegrenzungberchnen1/2(Filter) -> Memory/1
  Demux/2 -> Kommunikation_mit_GW1_3/7(RFID_Abmeldung)
  Demux/1 -> Kommunikation_mit_GW1_3/6(RFID_Anmeldung)
  Fifo Steuerung/2(Ziel_ereciht) -> Kommunikation_mit_GW1_3/5(ZielStation_Erreicht)
  Ziel anfordern/1 -> Kommunikation_mit_GW1_3/4(Ziel_anfordern)
  Fifo Steuerung/3("FifoArray ") -> Kommunikation_mit_GW1_3/3(FifoArray)
  UDPDaten_Aufteilen/4(RFID) -> Demux/1
  Auftrags_Koordination/3(Bearbeitet) -> Product/1
  Werkstueckerkannt1/1 -> Trafo/2(Winkel)
  BeobachterPos/1 -> Manual Switch/1
  Trafo/2(V_RobY) -> "VektorY "/1
  Trafo/1(V_RobX) -> VektorX/1
  Positionen_Robotinos_Filtern/1(RobPos) -> Manual Switch/2
  Memory2/1 -> Fehler_Merker/3(Transportbereich), Auftrags_Koordination/5(Transportbereich)
  Fifo Steuerung/1(ZielPos) -> Vektorberechnung/1(ZielPos)
  Vektorberechnung/1(Vektor) -> Vektorbrbegrenzungberchnen1/1(Vektor_In)
  Manual Switch/1 -> Fifo Steuerung/1(RobPos), Werkstueckerkannt1/1, Vektorbrbegrenzungberchnen1/4(RobPos), Vektorberechnung/2(RobotinoPos)
  Gain/1 -> Trafo/1(Vektor)
  Vektorbrbegrenzungberchnen1/1(Vektor) -> Gain/1
  Werkstueckerkannt/1 -> Fehler_Merker/4(Werkstueckerkannt), Auftrags_Koordination/4(Werkstueckerkannt)
  UDPDaten_Aufteilen/1(NeuerAuftrag) -> Auftrags_Koordination/1(NeuerAuftrag)
  Auftrags_Koordination/1(AktuellesZiel) -> Kommunikation_mit_GW1_3/1(Ziel), Fifo Steuerung/4(AktuellesZiel)
  UDPDaten_Aufteilen/3(ZielPos) -> Auftrags_Koordination/3(ZielPos)
  UDPDaten_Aufteilen/2(WerkstueckPos) -> Auftrags_Koordination/2(WerkstueckPos)
  RobotinoDaten1/1 -> UDPDaten_Aufteilen/1(UDP_GW1)
  Kommunikation_mit_GW1_3/1(Transportbereich) -> Memory2/1, Vektorbrbegrenzungberchnen1/3(Transportbereich_aktiv), Transportbereich_ein/aus/1
  Kommunikation_mit_GW1_3/2(Fertigungsbereich) -> Fertigungsbereich_ein/aus/1
  Kommunikation_mit_GW1_3/4(Aktion_an_Position) -> Aktion_an_Position/1
  Kommunikation_mit_GW1_3/3(Zielposition) -> Zielposition/1
  RobotinoDaten/1 -> Vektorberechnung/4(RobotinoDaten), Werkstueckerkannt/1
  Positionen_Robotinos_Filtern/2(StoerPos) -> Fifo Steuerung/2(StoerPos), Vektorberechnung/3(StoerPos)
  UDPDaten/1 -> Positionen_Robotinos_Filtern/1(UDPDaten)
  RobotinoID/1 -> Fifo Steuerung/3(RobotinoID), Positionen_Robotinos_Filtern/2(RobotinoID)
  Kommunikation_mit_GW1_3/5(Status) -> Memory3/1, Product/2
  Memory3/1 -> Auftrags_Koordination/6(Status)
  Auftrags_Koordination/2(Werkstueck) -> Kommunikation_mit_GW1_3/2(Werkstueck), Memory5/1
  Vektorberechnung/2(IRDaten) -> Vektorbrbegrenzungberchnen1/2(IRDaten)

== system Simulation_Robotinos/Subsystem ==
  Constant44 : Constant  Value=[0 0 ]
  Constant46 : Constant  Value=[2 1 1 1 7 1]
  Mux6 : Mux  Inputs=3
  Step : Step  Time=0.01  SampleTime=0
  Out1 : Outport
  wires:
  Constant46/1 -> Mux6/3
  Constant44/1 -> Mux6/1
  Mux6/1 -> Out1/1
  Step/1 -> Mux6/2

== system Simulation_Robotinos/Subsystem1 ==
  Constant44 : Constant  Value=[0 0 ]
  Constant46 : Constant  Value=[2 1 1 1 7 1]
  Mux6 : Mux  Inputs=3
  Step : Step  Time=0.01  SampleTime=0
  Out1 : Outport
  wires:
  Step/1 -> Mux6/2
  Mux6/1 -> Out1/1
  Constant44/1 -> Mux6/1
  Constant46/1 -> Mux6/3

== system Simulation_Robotinos/Subsystem2 ==
  Constant44 : Constant  Value=[0 0 ]
  Constant46 : Constant  Value=[2 1 1 1 7 1]
  Mux6 : Mux  Inputs=3
  Step : Step  Time=0.01  SampleTime=0
  Out1 : Outport
  wires:
  Constant46/1 -> Mux6/3
  Constant44/1 -> Mux6/1
  Mux6/1 -> Out1/1
  Step/1 -> Mux6/2

== system Simulation_Robotinos/Subsystem3 ==
  Constant44 : Constant  Value=[0 0 ]
  Constant46 : Constant  Value=[2 1 1 1 7 1]
  Mux6 : Mux  Inputs=3
  Step : Step  Time=0.01  SampleTime=0
  Out1 : Outport
  wires:
  Step/1 -> Mux6/2
  Mux6/1 -> Out1/1
  Constant44/1 -> Mux6/1
  Constant46/1 -> Mux6/3

== system Simulation_Robotinos/Subsystem4 ==
  Constant44 : Constant  Value=[0 0 ]
  Constant46 : Constant  Value=[2 1 1 1 7 1]
  Mux6 : Mux  Inputs=3
  Step : Step  Time=0.01  SampleTime=0
  Out1 : Outport
  wires:
  Constant46/1 -> Mux6/3
  Constant44/1 -> Mux6/1
  Mux6/1 -> Out1/1
  Step/1 -> Mux6/2

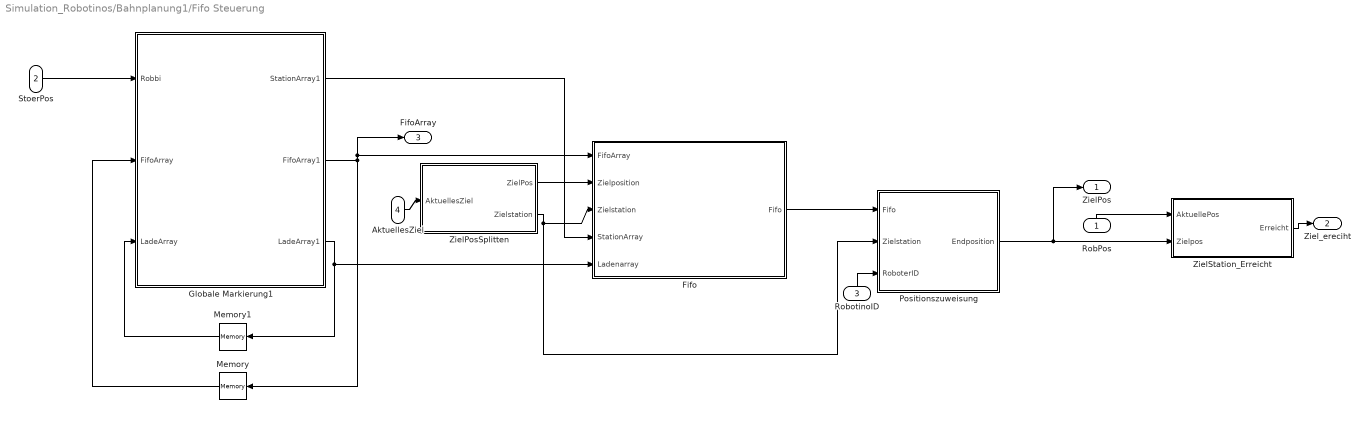
== system Simulation_Robotinos/Bahnplanung1/Fifo Steuerung ==
  RobPos : Inport  PortDimensions=3
  StoerPos : Inport  Port=2  PortDimensions=15
  RobotinoID : Inport  Port=3
  AktuellesZiel : Inport  Port=4
  Fifo : Stateflow chart  TreatAsAtomicUnit=on
  Globale Markierung1 : MATLAB Function  TreatAsAtomicUnit=on
  Memory : Memory
  Memory1 : Memory
  Positionszuweisung : MATLAB Function  TreatAsAtomicUnit=on
  ZielPosSplitten : MATLAB Function  TreatAsAtomicUnit=on
  ZielStation_Erreicht : MATLAB Function  TreatAsAtomicUnit=on
  ZielPos : Outport  PortDimensions=[1 2]
  Ziel_ereciht : Outport  Port=2
  "FifoArray " : Outport  Port=3
  wires:
  RobotinoID/1 -> Positionszuweisung/3(RoboterID)
  RobPos/1 -> ZielStation_Erreicht/1(AktuellePos)
  StoerPos/1 -> Globale Markierung1/1(Robbi)
  AktuellesZiel/1 -> ZielPosSplitten/1(AktuellesZiel)
  Positionszuweisung/1(Endposition) -> ZielStation_Erreicht/2(Zielpos), ZielPos/1
  Globale Markierung1/1(StationArray1) -> Fifo/4(StationArray)
  ZielPosSplitten/1(ZielPos) -> Fifo/2(Zielposition)
  ZielPosSplitten/2(Zielstation) -> Positionszuweisung/2(Zielstation), Fifo/3(Zielstation)
  Memory/1 -> Globale Markierung1/2(FifoArray)
  Globale Markierung1/3(LadeArray1) -> Fifo/5(Ladenarray), Memory1/1
  Memory1/1 -> Globale Markierung1/3(LadeArray)
  ZielStation_Erreicht/1(Erreicht) -> Ziel_ereciht/1
  Fifo/1(Fifo) -> Positionszuweisung/1(Fifo)
  Globale Markierung1/2(FifoArray1) -> "FifoArray "/1, Fifo/1(FifoArray), Memory/1

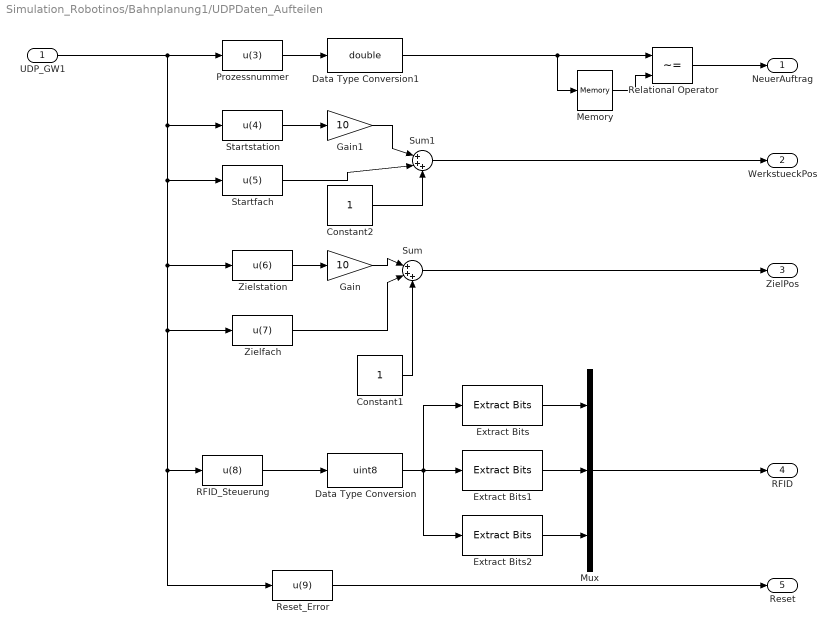
== system Simulation_Robotinos/Bahnplanung1/UDPDaten_Aufteilen ==
  UDP_GW1 : Inport
  Constant1 : Constant
  Constant2 : Constant
  Data Type Conversion : DataTypeConversion  OutDataTypeStr=uint8
  Data Type Conversion1 : DataTypeConversion  OutDataTypeStr=double
  Extract Bits : simulink/Logic and Bit Operations/Extract Bits  bitsToExtract=Range of bits  numBits=8  bitIdxRange=[0]  outScalingMode=Treat bit field as an integer
      settings: SourceProductName=Simulink
  Extract Bits1 : simulink/Logic and Bit Operations/Extract Bits  bitsToExtract=Range of bits  numBits=8  bitIdxRange=[1]  outScalingMode=Treat bit field as an integer
      settings: SourceProductName=Simulink
  Extract Bits2 : simulink/Logic and Bit Operations/Extract Bits  bitsToExtract=Range of bits  numBits=8  bitIdxRange=[2]  outScalingMode=Treat bit field as an integer
      settings: SourceProductName=Simulink
  Gain : Gain  Gain=10
  Gain1 : Gain  Gain=10
  Memory : Memory
  Mux : Mux  Inputs=3
  Prozessnummer : Fcn  Expr=u(3)
  RFID_Steuerung : Fcn  Expr=u(8)
  Relational Operator : RelationalOperator  Operator=~=  OutDataTypeStr=boolean  RndMeth=Nearest
  Reset_Error : Fcn  Expr=u(9)
  Startfach : Fcn  Expr=u(5)
  Startstation : Fcn  Expr=u(4)
  Sum : Sum  Inputs=|+++
  Sum1 : Sum  Inputs=|+++
  Zielfach : Fcn  Expr=u(7)
  Zielstation : Fcn  Expr=u(6)
  NeuerAuftrag : Outport
  WerkstueckPos : Outport  Port=2
  ZielPos : Outport  Port=3
  RFID : Outport  Port=4
  Reset : Outport  Port=5
  wires:
  Zielfach/1 -> Sum/2
  Gain/1 -> Sum/1
  Zielstation/1 -> Gain/1
  UDP_GW1/1 -> Prozessnummer/1, Startstation/1, Startfach/1, Zielstation/1, RFID_Steuerung/1, Reset_Error/1, Zielfach/1
  Sum1/1 -> WerkstueckPos/1
  Startfach/1 -> Sum1/2
  Gain1/1 -> Sum1/1
  Constant2/1 -> Sum1/3
  Startstation/1 -> Gain1/1
  Constant1/1 -> Sum/3
  Sum/1 -> ZielPos/1
  Relational Operator/1 -> NeuerAuftrag/1
  RFID_Steuerung/1 -> Data Type Conversion/1
  Data Type Conversion/1 -> Extract Bits2/1, Extract Bits1/1, Extract Bits/1
  Data Type Conversion1/1 -> Relational Operator/1, Memory/1
  Memory/1 -> Relational Operator/2
  Extract Bits1/1 -> Mux/2
  Mux/1 -> RFID/1
  Prozessnummer/1 -> Data Type Conversion1/1
  Extract Bits/1 -> Mux/1
  Extract Bits2/1 -> Mux/3
  Reset_Error/1 -> Reset/1

== system Simulation_Robotinos/Bahnplanung1/Vektorberechnung ==
  ZielPos : Inport
  RobotinoPos : Inport  Port=2
  StoerPos : Inport  Port=3
  RobotinoDaten : Inport  Port=4  PortDimensions=15
  AusweichVektorBerechnung : MATLAB Function  TreatAsAtomicUnit=on
  Ausweichmanoever : MATLAB Function  TreatAsAtomicUnit=on
  FahrendeRobotinosErkennen : MATLAB Function  TreatAsAtomicUnit=on
  Gain1 : Gain  Gain=-1
  IR_Daten_Erfassen : MATLAB Function  TreatAsAtomicUnit=on
  Memory : Memory
  Transport Delay : TransportDelay
  Vektorberechnung : MATLAB Function  TreatAsAtomicUnit=on
  Vektor : Outport
  IRDaten : Outport  Port=2
  wires:
  RobotinoPos/1 -> IR_Daten_Erfassen/2(RobPos), Vektorberechnung/3(RobotinoPos), AusweichVektorBerechnung/3(RobotinoPos), Ausweichmanoever/1(RobotinoPos)
  RobotinoDaten/1 -> IR_Daten_Erfassen/1(RobotinoDaten)
  StoerPos/1 -> Vektorberechnung/1(StoerPos), Ausweichmanoever/2(StoerPos), Transport Delay/1, FahrendeRobotinosErkennen/1(Stoerpos)
  ZielPos/1 -> Vektorberechnung/5(ZielPos), AusweichVektorBerechnung/2(ZielPos)
  Ausweichmanoever/1(Ausweich) -> AusweichVektorBerechnung/4(Ausweichwert)
  Vektorberechnung/1(Vektor) -> Gain1/1, AusweichVektorBerechnung/5(Vektor_In)
  Gain1/1 -> Ausweichmanoever/3(Vektor)
  IR_Daten_Erfassen/1(IRWerte) -> Vektorberechnung/2(IRWerte), IRDaten/1
  AusweichVektorBerechnung/1(Vektor) -> Vektor/1
  Vektorberechnung/2(Zone) -> Memory/1, AusweichVektorBerechnung/1(Zone)
  FahrendeRobotinosErkennen/1(Robotinofaehrt) -> Vektorberechnung/4(RobotinoFaehrt)
  Transport Delay/1 -> FahrendeRobotinosErkennen/2(Stoeralt)
  Memory/1 -> Vektorberechnung/6(AlteZone)

== system Simulation_Robotinos/Bahnplanung2/Fifo Steuerung ==
  RobPos : Inport  PortDimensions=3
  StoerPos : Inport  Port=2  PortDimensions=15
  RobotinoID : Inport  Port=3
  AktuellesZiel : Inport  Port=4
  Fifo : Stateflow chart  TreatAsAtomicUnit=on
  Globale Markierung1 : MATLAB Function  TreatAsAtomicUnit=on
  Memory : Memory
  Memory1 : Memory
  Positionszuweisung : MATLAB Function  TreatAsAtomicUnit=on
  ZielPosSplitten : MATLAB Function  TreatAsAtomicUnit=on
  ZielStation_Erreicht : MATLAB Function  TreatAsAtomicUnit=on
  ZielPos : Outport  PortDimensions=[1 2]
  Ziel_ereciht : Outport  Port=2
  "FifoArray " : Outport  Port=3
  wires:
  Globale Markierung1/2(FifoArray1) -> Memory/1, Fifo/1(FifoArray), "FifoArray "/1
  Fifo/1(Fifo) -> Positionszuweisung/1(Fifo)
  ZielStation_Erreicht/1(Erreicht) -> Ziel_ereciht/1
  Memory1/1 -> Globale Markierung1/3(LadeArray)
  Globale Markierung1/3(LadeArray1) -> Memory1/1, Fifo/5(Ladenarray)
  Memory/1 -> Globale Markierung1/2(FifoArray)
  ZielPosSplitten/2(Zielstation) -> Fifo/3(Zielstation), Positionszuweisung/2(Zielstation)
  ZielPosSplitten/1(ZielPos) -> Fifo/2(Zielposition)
  Globale Markierung1/1(StationArray1) -> Fifo/4(StationArray)
  Positionszuweisung/1(Endposition) -> ZielPos/1, ZielStation_Erreicht/2(Zielpos)
  AktuellesZiel/1 -> ZielPosSplitten/1(AktuellesZiel)
  StoerPos/1 -> Globale Markierung1/1(Robbi)
  RobPos/1 -> ZielStation_Erreicht/1(AktuellePos)
  RobotinoID/1 -> Positionszuweisung/3(RoboterID)

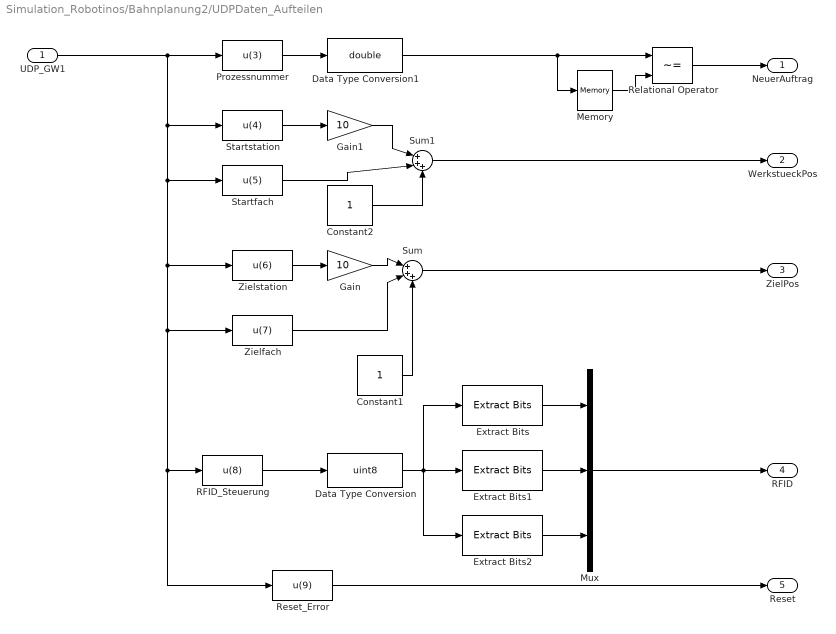
== system Simulation_Robotinos/Bahnplanung2/UDPDaten_Aufteilen ==
  UDP_GW1 : Inport
  Constant1 : Constant
  Constant2 : Constant
  Data Type Conversion : DataTypeConversion  OutDataTypeStr=uint8
  Data Type Conversion1 : DataTypeConversion  OutDataTypeStr=double
  Extract Bits : simulink/Logic and Bit Operations/Extract Bits  bitsToExtract=Range of bits  numBits=8  bitIdxRange=[0]  outScalingMode=Treat bit field as an integer
      settings: SourceProductName=Simulink
  Extract Bits1 : simulink/Logic and Bit Operations/Extract Bits  bitsToExtract=Range of bits  numBits=8  bitIdxRange=[1]  outScalingMode=Treat bit field as an integer
      settings: SourceProductName=Simulink
  Extract Bits2 : simulink/Logic and Bit Operations/Extract Bits  bitsToExtract=Range of bits  numBits=8  bitIdxRange=[2]  outScalingMode=Treat bit field as an integer
      settings: SourceProductName=Simulink
  Gain : Gain  Gain=10
  Gain1 : Gain  Gain=10
  Memory : Memory
  Mux : Mux  Inputs=3
  Prozessnummer : Fcn  Expr=u(3)
  RFID_Steuerung : Fcn  Expr=u(8)
  Relational Operator : RelationalOperator  Operator=~=  OutDataTypeStr=boolean  RndMeth=Nearest
  Reset_Error : Fcn  Expr=u(9)
  Startfach : Fcn  Expr=u(5)
  Startstation : Fcn  Expr=u(4)
  Sum : Sum  Inputs=|+++
  Sum1 : Sum  Inputs=|+++
  Zielfach : Fcn  Expr=u(7)
  Zielstation : Fcn  Expr=u(6)
  NeuerAuftrag : Outport
  WerkstueckPos : Outport  Port=2
  ZielPos : Outport  Port=3
  RFID : Outport  Port=4
  Reset : Outport  Port=5
  wires:
  Reset_Error/1 -> Reset/1
  Extract Bits2/1 -> Mux/3
  Extract Bits/1 -> Mux/1
  Prozessnummer/1 -> Data Type Conversion1/1
  Mux/1 -> RFID/1
  Extract Bits1/1 -> Mux/2
  Memory/1 -> Relational Operator/2
  Data Type Conversion1/1 -> Memory/1, Relational Operator/1
  Data Type Conversion/1 -> Extract Bits/1, Extract Bits1/1, Extract Bits2/1
  RFID_Steuerung/1 -> Data Type Conversion/1
  Relational Operator/1 -> NeuerAuftrag/1
  Sum/1 -> ZielPos/1
  Constant1/1 -> Sum/3
  Startstation/1 -> Gain1/1
  Constant2/1 -> Sum1/3
  Gain1/1 -> Sum1/1
  Startfach/1 -> Sum1/2
  Sum1/1 -> WerkstueckPos/1
  UDP_GW1/1 -> Zielfach/1, Reset_Error/1, RFID_Steuerung/1, Zielstation/1, Startfach/1, Startstation/1, Prozessnummer/1
  Zielstation/1 -> Gain/1
  Gain/1 -> Sum/1
  Zielfach/1 -> Sum/2

== system Simulation_Robotinos/Bahnplanung2/Vektorberechnung ==
  ZielPos : Inport
  RobotinoPos : Inport  Port=2
  StoerPos : Inport  Port=3
  RobotinoDaten : Inport  Port=4  PortDimensions=15
  AusweichVektorBerechnung : MATLAB Function  TreatAsAtomicUnit=on
  Ausweichmanoever : MATLAB Function  TreatAsAtomicUnit=on
  FahrendeRobotinosErkennen : MATLAB Function  TreatAsAtomicUnit=on
  Gain1 : Gain  Gain=-1
  IR_Daten_Erfassen : MATLAB Function  TreatAsAtomicUnit=on
  Memory : Memory
  Transport Delay : TransportDelay
  Vektorberechnung : MATLAB Function  TreatAsAtomicUnit=on
  Vektor : Outport
  IRDaten : Outport  Port=2
  wires:
  Memory/1 -> Vektorberechnung/6(AlteZone)
  Transport Delay/1 -> FahrendeRobotinosErkennen/2(Stoeralt)
  FahrendeRobotinosErkennen/1(Robotinofaehrt) -> Vektorberechnung/4(RobotinoFaehrt)
  Vektorberechnung/2(Zone) -> AusweichVektorBerechnung/1(Zone), Memory/1
  AusweichVektorBerechnung/1(Vektor) -> Vektor/1
  IR_Daten_Erfassen/1(IRWerte) -> IRDaten/1, Vektorberechnung/2(IRWerte)
  Gain1/1 -> Ausweichmanoever/3(Vektor)
  Vektorberechnung/1(Vektor) -> AusweichVektorBerechnung/5(Vektor_In), Gain1/1
  Ausweichmanoever/1(Ausweich) -> AusweichVektorBerechnung/4(Ausweichwert)
  ZielPos/1 -> AusweichVektorBerechnung/2(ZielPos), Vektorberechnung/5(ZielPos)
  StoerPos/1 -> FahrendeRobotinosErkennen/1(Stoerpos), Transport Delay/1, Ausweichmanoever/2(StoerPos), Vektorberechnung/1(StoerPos)
  RobotinoDaten/1 -> IR_Daten_Erfassen/1(RobotinoDaten)
  RobotinoPos/1 -> Ausweichmanoever/1(RobotinoPos), AusweichVektorBerechnung/3(RobotinoPos), Vektorberechnung/3(RobotinoPos), IR_Daten_Erfassen/2(RobPos)

== system Simulation_Robotinos/Bahnplanung3/Fifo Steuerung ==
  RobPos : Inport  PortDimensions=3
  StoerPos : Inport  Port=2  PortDimensions=15
  RobotinoID : Inport  Port=3
  AktuellesZiel : Inport  Port=4
  Fifo : Stateflow chart  TreatAsAtomicUnit=on
  Globale Markierung1 : MATLAB Function  TreatAsAtomicUnit=on
  Memory : Memory
  Memory1 : Memory
  Positionszuweisung : MATLAB Function  TreatAsAtomicUnit=on
  ZielPosSplitten : MATLAB Function  TreatAsAtomicUnit=on
  ZielStation_Erreicht : MATLAB Function  TreatAsAtomicUnit=on
  ZielPos : Outport  PortDimensions=[1 2]
  Ziel_ereciht : Outport  Port=2
  "FifoArray " : Outport  Port=3
  wires:
  RobotinoID/1 -> Positionszuweisung/3(RoboterID)
  RobPos/1 -> ZielStation_Erreicht/1(AktuellePos)
  StoerPos/1 -> Globale Markierung1/1(Robbi)
  AktuellesZiel/1 -> ZielPosSplitten/1(AktuellesZiel)
  Positionszuweisung/1(Endposition) -> ZielStation_Erreicht/2(Zielpos), ZielPos/1
  Globale Markierung1/1(StationArray1) -> Fifo/4(StationArray)
  ZielPosSplitten/1(ZielPos) -> Fifo/2(Zielposition)
  ZielPosSplitten/2(Zielstation) -> Positionszuweisung/2(Zielstation), Fifo/3(Zielstation)
  Memory/1 -> Globale Markierung1/2(FifoArray)
  Globale Markierung1/3(LadeArray1) -> Fifo/5(Ladenarray), Memory1/1
  Memory1/1 -> Globale Markierung1/3(LadeArray)
  ZielStation_Erreicht/1(Erreicht) -> Ziel_ereciht/1
  Fifo/1(Fifo) -> Positionszuweisung/1(Fifo)
  Globale Markierung1/2(FifoArray1) -> "FifoArray "/1, Fifo/1(FifoArray), Memory/1

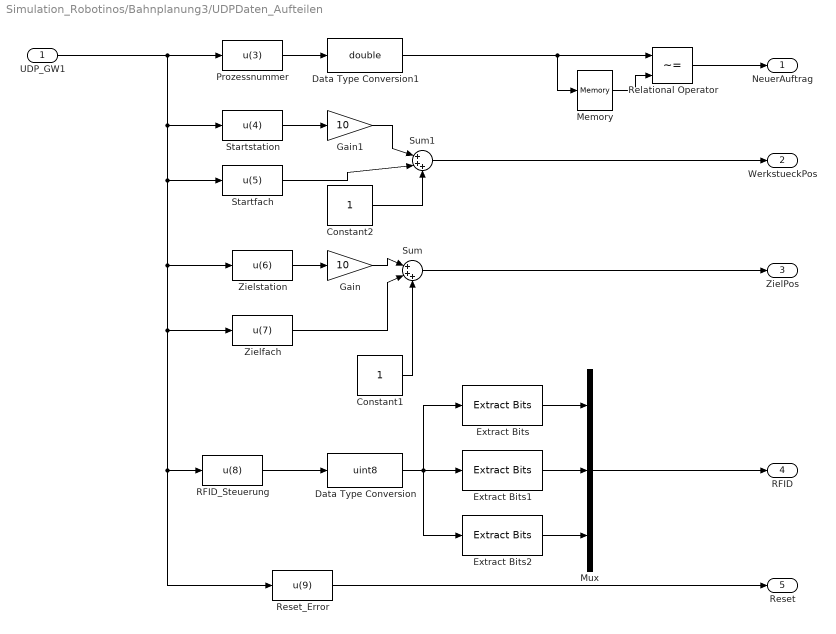
== system Simulation_Robotinos/Bahnplanung3/UDPDaten_Aufteilen ==
  UDP_GW1 : Inport
  Constant1 : Constant
  Constant2 : Constant
  Data Type Conversion : DataTypeConversion  OutDataTypeStr=uint8
  Data Type Conversion1 : DataTypeConversion  OutDataTypeStr=double
  Extract Bits : simulink/Logic and Bit Operations/Extract Bits  bitsToExtract=Range of bits  numBits=8  bitIdxRange=[0]  outScalingMode=Treat bit field as an integer
      settings: SourceProductName=Simulink
  Extract Bits1 : simulink/Logic and Bit Operations/Extract Bits  bitsToExtract=Range of bits  numBits=8  bitIdxRange=[1]  outScalingMode=Treat bit field as an integer
      settings: SourceProductName=Simulink
  Extract Bits2 : simulink/Logic and Bit Operations/Extract Bits  bitsToExtract=Range of bits  numBits=8  bitIdxRange=[2]  outScalingMode=Treat bit field as an integer
      settings: SourceProductName=Simulink
  Gain : Gain  Gain=10
  Gain1 : Gain  Gain=10
  Memory : Memory
  Mux : Mux  Inputs=3
  Prozessnummer : Fcn  Expr=u(3)
  RFID_Steuerung : Fcn  Expr=u(8)
  Relational Operator : RelationalOperator  Operator=~=  OutDataTypeStr=boolean  RndMeth=Nearest
  Reset_Error : Fcn  Expr=u(9)
  Startfach : Fcn  Expr=u(5)
  Startstation : Fcn  Expr=u(4)
  Sum : Sum  Inputs=|+++
  Sum1 : Sum  Inputs=|+++
  Zielfach : Fcn  Expr=u(7)
  Zielstation : Fcn  Expr=u(6)
  NeuerAuftrag : Outport
  WerkstueckPos : Outport  Port=2
  ZielPos : Outport  Port=3
  RFID : Outport  Port=4
  Reset : Outport  Port=5
  wires:
  Zielfach/1 -> Sum/2
  Gain/1 -> Sum/1
  Zielstation/1 -> Gain/1
  UDP_GW1/1 -> Prozessnummer/1, Startstation/1, Startfach/1, Zielstation/1, RFID_Steuerung/1, Reset_Error/1, Zielfach/1
  Sum1/1 -> WerkstueckPos/1
  Startfach/1 -> Sum1/2
  Gain1/1 -> Sum1/1
  Constant2/1 -> Sum1/3
  Startstation/1 -> Gain1/1
  Constant1/1 -> Sum/3
  Sum/1 -> ZielPos/1
  Relational Operator/1 -> NeuerAuftrag/1
  RFID_Steuerung/1 -> Data Type Conversion/1
  Data Type Conversion/1 -> Extract Bits2/1, Extract Bits1/1, Extract Bits/1
  Data Type Conversion1/1 -> Relational Operator/1, Memory/1
  Memory/1 -> Relational Operator/2
  Extract Bits1/1 -> Mux/2
  Mux/1 -> RFID/1
  Prozessnummer/1 -> Data Type Conversion1/1
  Extract Bits/1 -> Mux/1
  Extract Bits2/1 -> Mux/3
  Reset_Error/1 -> Reset/1

== system Simulation_Robotinos/Bahnplanung3/Vektorberechnung ==
  ZielPos : Inport
  RobotinoPos : Inport  Port=2
  StoerPos : Inport  Port=3
  RobotinoDaten : Inport  Port=4  PortDimensions=15
  AusweichVektorBerechnung : MATLAB Function  TreatAsAtomicUnit=on
  Ausweichmanoever : MATLAB Function  TreatAsAtomicUnit=on
  FahrendeRobotinosErkennen : MATLAB Function  TreatAsAtomicUnit=on
  Gain1 : Gain  Gain=-1
  IR_Daten_Erfassen : MATLAB Function  TreatAsAtomicUnit=on
  Memory : Memory
  Transport Delay : TransportDelay
  Vektorberechnung : MATLAB Function  TreatAsAtomicUnit=on
  Vektor : Outport
  IRDaten : Outport  Port=2
  wires:
  RobotinoPos/1 -> IR_Daten_Erfassen/2(RobPos), Vektorberechnung/3(RobotinoPos), AusweichVektorBerechnung/3(RobotinoPos), Ausweichmanoever/1(RobotinoPos)
  RobotinoDaten/1 -> IR_Daten_Erfassen/1(RobotinoDaten)
  StoerPos/1 -> Vektorberechnung/1(StoerPos), Ausweichmanoever/2(StoerPos), Transport Delay/1, FahrendeRobotinosErkennen/1(Stoerpos)
  ZielPos/1 -> Vektorberechnung/5(ZielPos), AusweichVektorBerechnung/2(ZielPos)
  Ausweichmanoever/1(Ausweich) -> AusweichVektorBerechnung/4(Ausweichwert)
  Vektorberechnung/1(Vektor) -> Gain1/1, AusweichVektorBerechnung/5(Vektor_In)
  Gain1/1 -> Ausweichmanoever/3(Vektor)
  IR_Daten_Erfassen/1(IRWerte) -> Vektorberechnung/2(IRWerte), IRDaten/1
  AusweichVektorBerechnung/1(Vektor) -> Vektor/1
  Vektorberechnung/2(Zone) -> Memory/1, AusweichVektorBerechnung/1(Zone)
  FahrendeRobotinosErkennen/1(Robotinofaehrt) -> Vektorberechnung/4(RobotinoFaehrt)
  Transport Delay/1 -> FahrendeRobotinosErkennen/2(Stoeralt)
  Memory/1 -> Vektorberechnung/6(AlteZone)

== system Simulation_Robotinos/Bahnplanung4/Fifo Steuerung ==
  RobPos : Inport  PortDimensions=3
  StoerPos : Inport  Port=2  PortDimensions=15
  RobotinoID : Inport  Port=3
  AktuellesZiel : Inport  Port=4
  Fifo : Stateflow chart  TreatAsAtomicUnit=on
  Globale Markierung1 : MATLAB Function  TreatAsAtomicUnit=on
  Memory : Memory
  Memory1 : Memory
  Positionszuweisung : MATLAB Function  TreatAsAtomicUnit=on
  ZielPosSplitten : MATLAB Function  TreatAsAtomicUnit=on
  ZielStation_Erreicht : MATLAB Function  TreatAsAtomicUnit=on
  ZielPos : Outport  PortDimensions=[1 2]
  Ziel_ereciht : Outport  Port=2
  "FifoArray " : Outport  Port=3
  wires:
  Globale Markierung1/2(FifoArray1) -> Memory/1, Fifo/1(FifoArray), "FifoArray "/1
  Fifo/1(Fifo) -> Positionszuweisung/1(Fifo)
  ZielStation_Erreicht/1(Erreicht) -> Ziel_ereciht/1
  Memory1/1 -> Globale Markierung1/3(LadeArray)
  Globale Markierung1/3(LadeArray1) -> Memory1/1, Fifo/5(Ladenarray)
  Memory/1 -> Globale Markierung1/2(FifoArray)
  ZielPosSplitten/2(Zielstation) -> Fifo/3(Zielstation), Positionszuweisung/2(Zielstation)
  ZielPosSplitten/1(ZielPos) -> Fifo/2(Zielposition)
  Globale Markierung1/1(StationArray1) -> Fifo/4(StationArray)
  Positionszuweisung/1(Endposition) -> ZielPos/1, ZielStation_Erreicht/2(Zielpos)
  AktuellesZiel/1 -> ZielPosSplitten/1(AktuellesZiel)
  StoerPos/1 -> Globale Markierung1/1(Robbi)
  RobPos/1 -> ZielStation_Erreicht/1(AktuellePos)
  RobotinoID/1 -> Positionszuweisung/3(RoboterID)
